simulink model "ex_sdl_flexible_shaft"  (R2022a)
settings: Solver=VariableStepAuto  StartTime=0.0  StopTime=stopTime  RelTol=1e-3  AbsTol=1e-6  EnableMultiTasking=on
InitFcn:
  | % Shaft properties
  | fShaft.Material = 'Aluminum Alloy';
  | fShaft.ShearModulus = 26E9;
  | fShaft.Diameter = 0.025;
  | fShaft.Length = 5;
  | fShaft.Density = 2.7E3;
  | fShaft.DampingCoeff = 0.02;
  | 
  | % Derived properties
  | fShaft.Stiffness = pi/32 * (fShaft.Diameter)^4 ...
  | * fShaft.ShearModulus / fShaft.Length;
  | 
  | fShaft.Inertia = pi/32 * (fShaft.Diameter)^4 ...
  | * fShaft.Density * fShaft.Length ;
values from neighbouring files (symbols this model uses):
  maxPressure = maxPressures(i)    [script1_generate_training_data.m]    (also in script3_test_model.m = maxPressuresTest(i))
undefined symbols (not defined in the file or in its folder): sigbuilder_block
libraries: fl_lib x12, nesl_utility x5, sdl_lib x3
CloseFcn:
  | try,close(h1_sdl_flexible_shaft),end
  | clear h1_sdl_flexible_shaft
  | try,close(h2_sdl_flexible_shaft),end
  | clear h2_sdl_flexible_shaft
  | 
  | 
  | clear simlog_sdl_flexible_shaft
Description:
  | Flexible Shaft
settings Model: FPTRunName=Active  Creator=The MathWorks, Inc.  LastModifiedBy=DNE
settings SolverCC: AutoScaleAbsTol=off  AlgebraicLoopSolver=TrustRegion  MaxZcPerStep=1
settings DataIOCC: LimitDataPoints=on  MaxDataPoints=10000  SaveFormat=Array  SignalLoggingName=logsout_sdl_flexible_shaft
settings OptimizationCC: ExpressionDepthLimit=2147483647  InitFltsAndDblsToZero=on  LifeSpan=inf
settings DebuggingCC: AlgebraicLoopMsg=none  SaveWithParameterizedLinksMsg=none  SignalResolutionControl=TryResolveAllWithWarning  MultiTaskDSMMsg=warning  MultiTaskCondExecSysMsg=none  UnconnectedInputMsg=warning  UnconnectedOutputMsg=warning  UnconnectedLineMsg=warning  StateNameClashWarn=warning  PregeneratedLibrarySubsystemCodeDiagnostic=none  SFUnexpectedBacktrackingDiag=warning  SFNoUnconditionalDefaultTransitionDiag=warning  SFExecutionAtInitializationDiag=none  SFMachineParentedDataDiag=warning  ArithmeticOperatorsInVariantConditions=warning
settings HardwareCC: ProdBitPerPointer=32  ProdBitPerSizeT=32  ProdBitPerPtrDiffT=32  ProdLargestAtomicFloat=None  ProdIntDivRoundTo=Undefined  ProdEndianess=Unspecified  ProdWordSize=32  ProdHWDeviceType=32-bit Generic  TargetBitPerPointer=64  TargetBitPerSizeT=64  TargetBitPerPtrDiffT=64  TargetLongLongMode=on  TargetIntDivRoundTo=Zero  TargetEndianess=LittleEndian  TargetWordSize=64  TargetHWDeviceType=MATLAB Host  ProdEqTarget=off
settings ModelReferenceCC: PropagateSignalLabelsOutOfModel=off
settings SFSimCC: SimUseLocalCustomCode=off  CustomCodeUndefinedFunction=UseInterfaceOnly
settings RTWCC: Description=Generic Real-Time Target  RTWUseLocalCustomCode=off  DLArmComputeVersion=19.05
settings CodeAppCC: StateflowObjectComments=on
settings GRTTargetCC: TargetLangStandard=C89/C90 (ANSI)  CombineOutputUpdateFcns=off  GRTInterface=on
settings ConfigComp: CovMetricSettings=dw  CovSaveCumulativeToWorkspaceVar=on  CovSaveSingleToWorkspaceVar=on  CovExternalEMLEnable=off
settings SimscapeCC: SimscapeLogType=all  SimscapeLogSimulationStatistics=on  SimscapeLogName=simlog_sdl_flexible_shaft  SimscapeLogDataHistory=10000

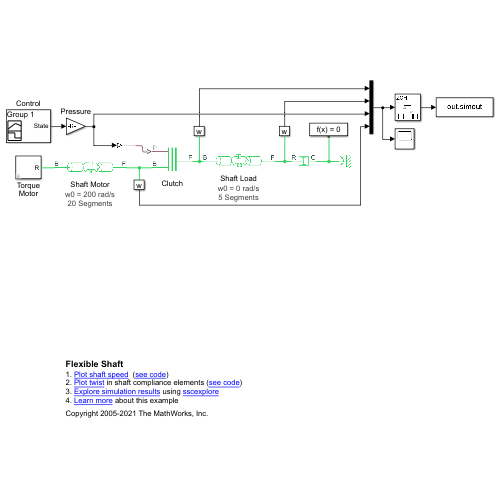
[thumbnail: Simulink's stored preview of the top-level diagram]
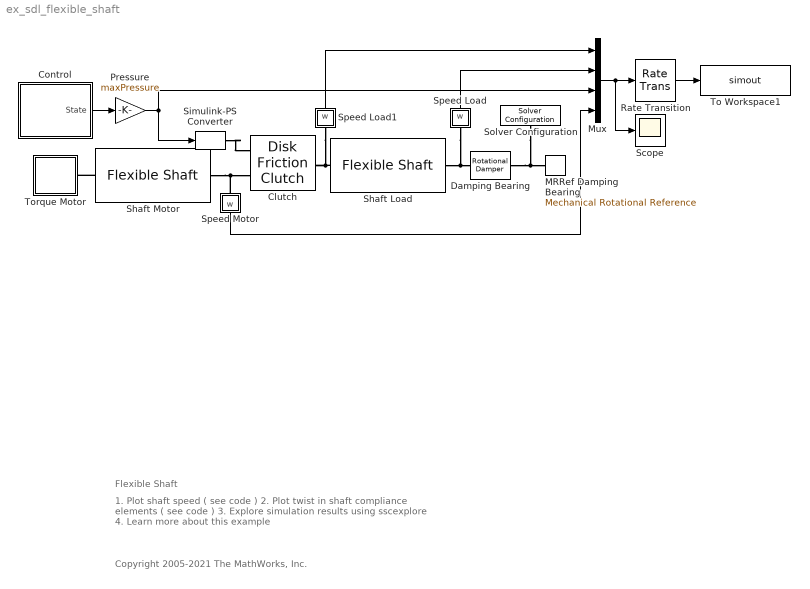
== system ex_sdl_flexible_shaft ==
  note: Flexible Shaft
  note: 1. Plot shaft speed ( see code )
      | 2. Plot twist in shaft compliance elements ( see code )
      | 3. Explore simulation results using sscexplore
      | 4. Learn more about this example
  note: Copyright 2005-2021 The MathWorks, Inc.
  Clutch : sdl_lib/Clutches/Disk Friction Clutch  geometry_model=1  r_eff=40 mm  d_o=150 mm  d_i=100 mm  nS=6  piston_area=0.001 m^2  unidirectional=0  friction_model=1  mu_w_vector=[ 0 0.1 0.2 0.3 0.4 0.5 1 2 5 10 100 1000 ] rad/s  temperature_TLU=[280.0, 300.0, 320.0] K  mu_static=1.1  mu_static_vector=[0.4, 0.38, 0.36]  mu_coulomb=1  mu_coulomb_vector=[ 0.29 0.28 0.26 0.22 0.21 0.2 0.2 0.19 0.19 0.19 0.19 0.19 ]  mu_coulomb_temp_vector=[0.3, 0.28, 0.25]  mu_coulomb_matrix=[0.34, 0.32, 0.3; 0.3, 0.28, 0.25; 0.25, 0.2, 0.15]  mu_interp_method=1  mu_extrap_method=1  d_f=1  w_tol=0.001 rad/s  pressure_min=0 Pa  mu_visc=0 N*m/(rad/s)  initial_state_locked=0  enable_faults=simscape.enum.onoff.off  fault_type=sdl.enum.clutchFault.lock  external_fault=simscape.enum.onoff.off  temporal_fault=simscape.enum.onoff.off  fault_time=5 s  report_fault=simscape.enum.assert.action.none  thermal_mass=25 kJ/K  T_init=300 K
      settings: SourceProductBaseCode=LD  InternalSimscapePortConfiguration="{\"Bottom\":[],\"Left\":[{\"id\":\"P\",\"label\":\"P\",\"type\":\"input\"},{\"id\":\"B\",\"label\":\"B\",\"type\":\"foundation.mechanical.rotational.rotational\"}],\"Right\":[{\"id\":\"F\",\"label\":\"F\",\"type\":\"foundation.mechanical.rotational.rotational\"}],\"Top\":[]}"
  Control : Subsystem  Tag=STV Subsys  LoadFcn=sigbuilder_block('load');  StartFcn=sigbuilder_block('start');  StopFcn=sigbuilder_block('stop');  ClipboardFcn=sigbuilder_block('clipboard');  mask(Sigbuilder block){tuvar=[0:10]}
      mask help: Sigbuilder GUI
      mask init:
      | if ~strcmp(get_param(bdroot(gcbh),'SimulationStatus'),'stopped') tuvar = sigbuilder_block('maskInit'); end
      settings: CopyFcn=sigbuilder_block('copy');  DeleteFcn=sigbuilder_block('delete');  ModelCloseFcn=sigbuilder_block('modelClose');  PreSaveFcn=sigbuilder_block('preSave');  PauseFcn=sigbuilder_block('pause')  ContinueFcn=sigbuilder_block('continue')  NameChangeFcn=sigbuilder_block('namechange');  OpenFcn=sigbuilder_block('open',[320.25 141 457.5 466.5 ]);  CloseFcn=sigbuilder_block('close');
      mask Display: plot(0, 0, 100, 100,[2, 2, 32, 32, 2], [68, 8, 8, 68, 68],[32, 2], [38, 38], [32, 19, 2],[53, 60, 44], [32, 17, 17, 2],[16, 16, 31, 31]);txt = getActiveGroup(gcbh);text(2, 100, txt,'verticalAlignment', 'top');
  Damping Bearing : fl_lib/Mechanical/Rotational Elements/Rotational Damper  D=0.01 N*m/(rad/s)  w_specify=off  w_priority=High  w=0 rad/s  w_nominal_specify=off  w_nominal_unit=rad/s  w_nominal_value=1  t_specify=off  t_priority=High  t=0 N*m  t_nominal_specify=off  t_nominal_unit=N*m  t_nominal_value=1
      settings: SourceProductBaseCode=PW,SS,VE
  MRRef Damping Bearing : fl_lib/Mechanical/Rotational Elements/Mechanical Rotational Reference
      settings: SourceProductBaseCode=PW,SS,VE
  Mux : Mux
  Pressure : Gain  Gain=maxPressure  SaturateOnIntegerOverflow=on  OutDataTypeStr=Inherit: Same as input  ParamDataTypeStr=Inherit: Same as input
  Rate Transition : RateTransition  OutPortSampleTime=timeInterval
  Scope : Scope
  Shaft Load : sdl_lib/Couplings & Drives/Flexible Shaft  modelTransverse=simscape.enum.onoff.off  n_segments=5  parameterization=sdl.enum.shaftParameterization.StiffnessInertia  length=fShaft.Length m  lengths=[1, .5, .25] m  shaft_stiffness=fShaft.Stiffness N*m/rad  shaft_inertia=fShaft.Inertia kg*m^2  shaft_stiffnesses=[400000, 200000, 100000] N*m/rad  shaft_inertias=[.025, .02, .015] kg*m^2  eiIN=5e5 m^4*Pa  rhoaIN=19 kg/m  eiINs=[600000, 500000, 400000] m^4*Pa  rhoaINs=[20, 19, 18] kg/m  density=fShaft.Density kg/m^3  shear_modulus=fShaft.ShearModulus Pa  elastic_modulus=200e9 Pa  shaft_construction=sdl.enum.shaftConstruction.solid  diameter_outer=fShaft.Diameter m  diameter_inner=fShaft.Diameter/2 m  diameter_outers=[.085, .075, .065] m  diameter_inners=[.055, .05, .045] m  damping_ratio=fShaft.DampingCoeff  mu_visc_BF=[0, 0] N*m/(rad/s)  mu_visc=[ 0 0 ] N*m/(rad/s)  initial_deflection=0 rad  initial_velocity=0 rad/s  num_supports=sdl.enum.num_supports.two  z_support=[0, fShaft.Length] m  boundaryB1=sdl.enum.shaftSupport.clamp  DrotB1_row=[100000, 100000] N*m/(rad/s)  DtransB1_row=[200000, -440000, -440000, 3500000] N/(m/s)  DtransB1_w_mat=[200000, -440000, -440000, 3500000; 100000, -250000, -250000, 1400000; 50000, -100000, -100000, 200000] N/(m/s)  KrotB1_row=[10000000, 10000000] N*m/rad  KtransB1_row=[10000000, -2000000, -3000000, 50000000] N/m  KtransB1_w_mat=[10000000, -6000000, -35000000, 80000000; 10000000, -2000000, -3000000, 50000000; 10000000, -500000, -25000000, 30000000] N/m  boundaryI1=sdl.enum.shaftSupport.clamp  DrotI1_row=[100000, 100000] N*m/(rad/s)  DtransI1_row=[200000, -440000, -440000, 3500000] N/(m/s)  DtransI1_w_mat=[200000, -440000, -440000, 3500000; 100000, -250000, -250000, 1400000; 50000, -100000, -100000, 200000] N/(m/s)  KrotI1_row=[10000000, 10000000] N*m/rad  KtransI1_row=[10000000, -2000000, -3000000, 50000000] N/m  KtransI1_w_mat=[10000000, -6000000, -35000000, 80000000; 10000000, -2000000, -3000000, 50000000; 10000000, -500000, -25000000, 30000000] N/m  boundaryI2=sdl.enum.shaftSupport.clamp  DrotI2_row=[100000, 100000] N*m/(rad/s)  DtransI2_row=[200000, -440000, -440000, 3500000] N/(m/s)  DtransI2_w_mat=[200000, -440000, -440000, 3500000; 100000, -250000, -250000, 1400000; 50000, -100000, -100000, 200000] N/(m/s)  KrotI2_row=[10000000, 10000000] N*m/rad  KtransI2_row=[10000000, -2000000, -3000000, 50000000] N/m  KtransI2_w_mat=[10000000, -6000000, -35000000, 80000000; 10000000, -2000000, -3000000, 50000000; 10000000, -500000, -25000000, 30000000] N/m  boundaryF1=sdl.enum.shaftSupport.clamp  DrotF1_row=[100000, 100000] N*m/(rad/s)  DtransF1_row=[200000, -440000, -440000, 3500000] N/(m/s)  DtransF1_w_mat=[200000, -440000, -440000, 3500000; 100000, -250000, -250000, 1400000; 50000, -100000, -100000, 200000] N/(m/s)  KrotF1_row=[10000000, 10000000] N*m/rad  KtransF1_row=[10000000, -2000000, -3000000, 50000000] N/m  KtransF1_w_mat=[10000000, -6000000, -35000000, 80000000; 10000000, -2000000, -3000000, 50000000; 10000000, -500000, -25000000, 30000000] N/m  bearing_speed=[200, 500, 1500] rpm  alpha=10 1/s  beta=1e-8 s  noDisk=sdl.enum.shaftDisks.none  zDisk=0.5 m  mDiskIN=2 kg  IdDiskIN=0.025 kg*m^2  IpDiskIN=0.050 kg*m^2  offsetMR=[.01, .01] m*kg  offsetMassLocation=[.33, .67] m  offsetMR_initialAngleIN=[0, pi] rad  AnalysisMethod=sdl.enum.bendingAnalysisMethod.LumpedMass  ModeInputMethod=sdl.enum.modeInputMethod.SimscapeDetermined  numModesIn=6  mode_speed_dependency=sdl.enum.mode_speed_dependency.Static  OmegaNom=100 rpm  wMax=50000 rad/s  dz=0.01 m  userMode_w=[280, 644, 615, 1285] rad/s  userMode_w_mat=[257, 780, 580, 1560; 280, 644, 615, 1285; 294, 513, 636, 1020] rad/s  userMode_z=[0, .1, .2, .3, .4, .5, .6, .7, .8, .9, 1] m  userMode_shapeX=[.1648, .0086, -.2759, .0162; .1671, .0093, -.2231, .0133; .1691, .01, -.1689, .0102; .1707, .0105, -.1135, .007; .1717, .0108, -.057, .0035; .1721, .0109, 0, 0; .1717, .0108, .057, -.0035; .1707, .0105, .1135, -.007; .1691, .01, .1689, -.0102; .1671, .0093, .2231, -.0133; .1648, .0086, .2759, -.0162]  userMode_shapeX_mat=cat(3, [.1842, .0134, -.3072, .0272; .1863, .0152, -.2482, .0226; .1882, .0169, -.1878, .0176; .1897, .0182, -.1261, .0121; .1906, .019, -.0634, .0062; .191, .0193, 0, 0; .1906, .019, .0634, -.0062; .1897, .0182, .1261, -.0121; .1882, .0169, .1878, -.0176; .1863, .0152, .2482, -.0226; .1842, .0134, .3072, -.0272], [.1648, .0086, -.2759, .0162; .1671, .0093, -.2231, .0133; .1691, .01, -.1689, .0102; .1707, .0105, -.1135, .007; .1717, .0108, -.057, .0035; .1721, .0109, 0, 0; .1717, .0108, .057, -.0035; .1707, .0105, .1135, -.007; .1691, .01, .1689, -.0102; .1671, .0093, .2231, -.0133; .1648, .0086, .2759, -.0162], [.1291, .0046, -.2166, .0082; .131, .0048, -.1751, .0067; .1327, .005, -.1327, .0051; .1341, .0052, -.0891, .0035; .135, .0053, -.0448, .0017; .1353, .0053, 0, 0; .135, .0053, .0448, -.0017; .1341, .0052, .0891, -.0035; .1327, .005, .1327, -.0051; .131, .0048, .1751, -.0067; .1291, .0046, .2166, -.0082])  userMode_shapeY=[.1193, -.1784, -.1997, -.3348; .1209, -.1933, -.1615, -.2751; .1224, -.2068, -.1223, -.2119; .1235, -.2176, -.0821, -.1445; .1243, -.2245, -.0413, -.0734; .1246, -.2269, 0, 0; .1243, -.2245, .0413, .0734; .1235, -.2176, .0821, .1445; .1224, -.2068, .1223, .2119; .1209, -.1933, .1615, .2751; .1193, -.1784, .1997, .3348]  userMode_shapeY_mat=cat(3, [.0885, -.1625, -.1475, -.3301; .0895, -.1847, -.1192, -.2745; .0904, -.2048, -.0902, -.2141; .0911, -.2209, -.0606, -.1475; .0916, -.2313, -.0304, -.0754; .0917, -.2349, 0, 0; .0916, -.2313, .0304, .0754; .0911, -.2209, .0606, .1475; .0904, -.2048, .0902, .2141; .0895, -.1847, .1192, .2745; .0885, -.1625, .1475, .3301], [.1193, -.1784, -.1997, -.3348; .1209, -.1933, -.1615, -.2751; .1224, -.2068, -.1223, -.2119; .1235, -.2176, -.0821, -.1445; .1243, -.2245, -.0413, -.0734; .1246, -.2269, 0, 0; .1243, -.2245, .0413, .0734; .1235, -.2176, .0821, .1445; .1224, -.2068, .1223, .2119; .1209, -.1933, .1615, .2751; .1193, -.1784, .1997, .3348], [.1566, -.1901, -.2628, -.3377; .1589, -.1994, -.2125, -.2753; .161, -.2079, -.1609, -.2103; .1627, -.2146, -.1081, -.1424; .1638, -.219, -.0544, -.0719; .1642, -.2205, 0, 0; .1638, -.219, .0544, .0719; .1627, -.2146, .1081, .1424; .161, -.2079, .1609, .2103; .1589, -.1994, .2125, .2753; .1566, -.1901, .2628, .3377])
      settings: SourceProductBaseCode=LD  InternalSimscapePortConfiguration="{\"Bottom\":[],\"Left\":[{\"id\":\"B\",\"label\":\"B\",\"type\":\"foundation.mechanical.rotational.rotational\"}],\"Right\":[{\"id\":\"F\",\"label\":\"F\",\"type\":\"foundation.mechanical.rotational.rotational\"}],\"Top\":[]}"
      settings: AttributesFormatString=|
      | w0 = %<initial_velocity> %<initial_velocity_unit>
      | %<n_segments> Segments
  Shaft Motor : sdl_lib/Couplings & Drives/Flexible Shaft  modelTransverse=simscape.enum.onoff.off  n_segments=20  parameterization=sdl.enum.shaftParameterization.MaterialProperties  length=fShaft.Length m  lengths=[1, .5, .25] m  shaft_stiffness=fShaft.Stiffness N*m/rad  shaft_inertia=fShaft.Inertia kg*m^2  shaft_stiffnesses=[400000, 200000, 100000] N*m/rad  shaft_inertias=[.025, .02, .015] kg*m^2  eiIN=5e5 m^4*Pa  rhoaIN=19 kg/m  eiINs=[600000, 500000, 400000] m^4*Pa  rhoaINs=[20, 19, 18] kg/m  density=fShaft.Density kg/m^3  shear_modulus=fShaft.ShearModulus Pa  elastic_modulus=200e9 Pa  shaft_construction=sdl.enum.shaftConstruction.annular  diameter_outer=fShaft.Diameter m  diameter_inner=fShaft.Diameter/2 m  diameter_outers=[.085, .075, .065] m  diameter_inners=[.055, .05, .045] m  damping_ratio=fShaft.DampingCoeff  mu_visc_BF=[0, 0] N*m/(rad/s)  mu_visc=[ 0 0 ] N*m/(rad/s)  initial_deflection=0 rad  initial_velocity=200 rad/s  num_supports=sdl.enum.num_supports.two  z_support=[0, fShaft.Length] m  boundaryB1=sdl.enum.shaftSupport.clamp  DrotB1_row=[1000, 1000] N*m/(rad/s)  DtransB1_row=[20000, -44000, -44000, 350000] N/(m/s)  DtransB1_w_mat=[200000, -440000, -440000, 3500000; 100000, -250000, -250000, 1400000; 50000, -100000, -100000, 200000] N/(m/s)  KrotB1_row=[10000, 10000] N*m/rad  KtransB1_row=[1000000, -200000, -300000, 5000000] N/m  KtransB1_w_mat=[10000000, -6000000, -35000000, 80000000; 10000000, -2000000, -3000000, 50000000; 10000000, -500000, -25000000, 30000000] N/m  boundaryI1=sdl.enum.shaftSupport.clamp  DrotI1_row=[100000, 100000] N*m/(rad/s)  DtransI1_row=[200000, -440000, -440000, 3500000] N/(m/s)  DtransI1_w_mat=[200000, -440000, -440000, 3500000; 100000, -250000, -250000, 1400000; 50000, -100000, -100000, 200000] N/(m/s)  KrotI1_row=[10000000, 10000000] N*m/rad  KtransI1_row=[10000000, -2000000, -3000000, 50000000] N/m  KtransI1_w_mat=[10000000, -6000000, -35000000, 80000000; 10000000, -2000000, -3000000, 50000000; 10000000, -500000, -25000000, 30000000] N/m  boundaryI2=sdl.enum.shaftSupport.clamp  DrotI2_row=[100000, 100000] N*m/(rad/s)  DtransI2_row=[200000, -440000, -440000, 3500000] N/(m/s)  DtransI2_w_mat=[200000, -440000, -440000, 3500000; 100000, -250000, -250000, 1400000; 50000, -100000, -100000, 200000] N/(m/s)  KrotI2_row=[10000000, 10000000] N*m/rad  KtransI2_row=[10000000, -2000000, -3000000, 50000000] N/m  KtransI2_w_mat=[10000000, -6000000, -35000000, 80000000; 10000000, -2000000, -3000000, 50000000; 10000000, -500000, -25000000, 30000000] N/m  boundaryF1=sdl.enum.shaftSupport.clamp  DrotF1_row=[1000, 1000] N*m/(rad/s)  DtransF1_row=[20000, -44000, -44000, 350000] N/(m/s)  DtransF1_w_mat=[200000, -440000, -440000, 3500000; 100000, -250000, -250000, 1400000; 50000, -100000, -100000, 200000] N/(m/s)  KrotF1_row=[10000, 10000] N*m/rad  KtransF1_row=[1000000, -200000, -300000, 5000000] N/m  KtransF1_w_mat=[10000000, -6000000, -35000000, 80000000; 10000000, -2000000, -3000000, 50000000; 10000000, -500000, -25000000, 30000000] N/m  bearing_speed=[200, 500, 1500] rpm  alpha=10 1/s  beta=1e-8 s  noDisk=sdl.enum.shaftDisks.none  zDisk=0.5 m  mDiskIN=2 kg  IdDiskIN=0.025 kg*m^2  IpDiskIN=0.050 kg*m^2  offsetMR=[.01, .01] m*kg  offsetMassLocation=[.33, .67] m  offsetMR_initialAngleIN=[0, pi] rad  AnalysisMethod=sdl.enum.bendingAnalysisMethod.LumpedMass  ModeInputMethod=sdl.enum.modeInputMethod.SimscapeDetermined  numModesIn=6  mode_speed_dependency=sdl.enum.mode_speed_dependency.Static  OmegaNom=100 rpm  wMax=50000 rad/s  dz=0.01 m  userMode_w=[162, 162, 649, 649, 1460, 1460, 2596, 2596] rad/s  userMode_w_mat=[257, 780, 580, 1560; 280, 644, 615, 1285; 294, 513, 636, 1020] rad/s  userMode_z=[0, .1, .2, .3, .4, .5, .6, .7, .8, .9, 1] m  userMode_shapeX=[.1648, .0086, -.2759, .0162; .1671, .0093, -.2231, .0133; .1691, .01, -.1689, .0102; .1707, .0105, -.1135, .007; .1717, .0108, -.057, .0035; .1721, .0109, 0, 0; .1717, .0108, .057, -.0035; .1707, .0105, .1135, -.007; .1691, .01, .1689, -.0102; .1671, .0093, .2231, -.0133; .1648, .0086, .2759, -.0162]  userMode_shapeX_mat=cat(3, [.1842, .0134, -.3072, .0272; .1863, .0152, -.2482, .0226; .1882, .0169, -.1878, .0176; .1897, .0182, -.1261, .0121; .1906, .019, -.0634, .0062; .191, .0193, 0, 0; .1906, .019, .0634, -.0062; .1897, .0182, .1261, -.0121; .1882, .0169, .1878, -.0176; .1863, .0152, .2482, -.0226; .1842, .0134, .3072, -.0272], [.1648, .0086, -.2759, .0162; .1671, .0093, -.2231, .0133; .1691, .01, -.1689, .0102; .1707, .0105, -.1135, .007; .1717, .0108, -.057, .0035; .1721, .0109, 0, 0; .1717, .0108, .057, -.0035; .1707, .0105, .1135, -.007; .1691, .01, .1689, -.0102; .1671, .0093, .2231, -.0133; .1648, .0086, .2759, -.0162], [.1291, .0046, -.2166, .0082; .131, .0048, -.1751, .0067; .1327, .005, -.1327, .0051; .1341, .0052, -.0891, .0035; .135, .0053, -.0448, .0017; .1353, .0053, 0, 0; .135, .0053, .0448, -.0017; .1341, .0052, .0891, -.0035; .1327, .005, .1327, -.0051; .131, .0048, .1751, -.0067; .1291, .0046, .2166, -.0082])  userMode_shapeY=[.1193, -.1784, -.1997, -.3348; .1209, -.1933, -.1615, -.2751; .1224, -.2068, -.1223, -.2119; .1235, -.2176, -.0821, -.1445; .1243, -.2245, -.0413, -.0734; .1246, -.2269, 0, 0; .1243, -.2245, .0413, .0734; .1235, -.2176, .0821, .1445; .1224, -.2068, .1223, .2119; .1209, -.1933, .1615, .2751; .1193, -.1784, .1997, .3348]  userMode_shapeY_mat=cat(3, [.0885, -.1625, -.1475, -.3301; .0895, -.1847, -.1192, -.2745; .0904, -.2048, -.0902, -.2141; .0911, -.2209, -.0606, -.1475; .0916, -.2313, -.0304, -.0754; .0917, -.2349, 0, 0; .0916, -.2313, .0304, .0754; .0911, -.2209, .0606, .1475; .0904, -.2048, .0902, .2141; .0895, -.1847, .1192, .2745; .0885, -.1625, .1475, .3301], [.1193, -.1784, -.1997, -.3348; .1209, -.1933, -.1615, -.2751; .1224, -.2068, -.1223, -.2119; .1235, -.2176, -.0821, -.1445; .1243, -.2245, -.0413, -.0734; .1246, -.2269, 0, 0; .1243, -.2245, .0413, .0734; .1235, -.2176, .0821, .1445; .1224, -.2068, .1223, .2119; .1209, -.1933, .1615, .2751; .1193, -.1784, .1997, .3348], [.1566, -.1901, -.2628, -.3377; .1589, -.1994, -.2125, -.2753; .161, -.2079, -.1609, -.2103; .1627, -.2146, -.1081, -.1424; .1638, -.219, -.0544, -.0719; .1642, -.2205, 0, 0; .1638, -.219, .0544, .0719; .1627, -.2146, .1081, .1424; .161, -.2079, .1609, .2103; .1589, -.1994, .2125, .2753; .1566, -.1901, .2628, .3377])
      settings: SourceProductBaseCode=LD  InternalSimscapePortConfiguration="{\"Bottom\":[],\"Left\":[{\"id\":\"B\",\"label\":\"B\",\"type\":\"foundation.mechanical.rotational.rotational\"}],\"Right\":[{\"id\":\"F\",\"label\":\"F\",\"type\":\"foundation.mechanical.rotational.rotational\"}],\"Top\":[]}"
      settings: AttributesFormatString=|
      | w0 = %<initial_velocity> %<initial_velocity_unit>
      | %<n_segments> Segments
  Simulink-PS Converter : nesl_utility/Simulink-PS Converter  PhysicalDomain=network_engine_domain  SubClassName=ps_input  LeftPortType=input  RightPortType=output  PseudoPeriodic=off  Frequencies=[]  NoiseDistribution=none  NoiseParameters=[]  Unit=Pa  AffineConversion=off  FilteringAndDerivatives=zero  SimscapeFilterOrder=1  InputFilterTimeConstant=.001  UdotUserProvided=0
      settings: SourceProductBaseCode=SS,PW,VE
  Solver Configuration : nesl_utility/Solver Configuration  PhysicalDomain=network_engine_domain  SubClassName=solver  LeftPortType=input  RightPortType=generic  Tones=[]  Harmonics=[]  SimulateNoise=off  Profile=off  UseLocalSampling=off  EnableSwitchedLinearOptims=on  FrequencyDomain=off  UseCCode=off  RelTol=0.001  AbsTol=1e-06  MinStep=1e-09  ToWorkspace=off  RevertToSquareIcSolve=off  NumHomotopyIterations=100  PhasorMode=off  PhasorModeNumHarmonics=1  IndexReductionMethod=DerivativeReplacement  DoDC=off  ResidualTolerance=1e-9  UseLocalSolver=off  LocalSolverChoice=NE_PARTITIONING_ADVANCER  LocalSolverSampleTime=.0001  DoFixedCost=off  MaxNonlinIter=3  MaxModeIter=2  ComputeImpulses=off  ImpulseIterations=2  LinearAlgebra=auto  LinearAlgebraNumThread=0  EquationFormulation=NE_TIME_EF  DelaysMemoryBudget=1024  AutomaticFiltering=on  FilteringTimeConstant=0.001  PartitionStorageMethod=EXHAUSTIVE  PartitionMemoryBudget=1024  PartitionMethod=ROBUST
      settings: SourceProductBaseCode=SS,PW,VE
  Speed Load : Subsystem
      mask Display: disp('w')
  Speed Load1 : Subsystem
      mask Display: disp('w')
  Speed Motor : Subsystem
      mask Display: disp('w')
  To Workspace1 : ToWorkspace  VariableName=simout  SaveFormat=Timeseries  SampleTime=-1
  Torque Motor : Subsystem  mask(Constant Torque Motor){motorTorque=20, bearingD=0.1}
      mask prompts: motorTorque "Demanded torque (Nm)"; bearingD "Bearing damping ( Nm/(rad/s) )"
      mask help:
      | Models a simple constant torque motor with bearing loss.
      |
      | OutputTorque = DemandedTorque - BearingDamping * RotationalSpeed
  wires:
  Pressure/1 -> Mux/3, Simulink-PS Converter/1
  Mux/1 -> Scope/1, Rate Transition/1
  Rate Transition/1 -> To Workspace1/1
  Speed Load1/1(w) -> Mux/1
  Speed Load/1(w) -> Mux/2
  Control/1(State) -> Pressure/1
  Speed Motor/1(w) -> Mux/4
  connections:
  Shaft Motor/LConn1 -- Torque Motor/LConn1
  Shaft Load/RConn1 -- Speed Load/LConn1 -- Damping Bearing/LConn1
  Damping Bearing/RConn1 -- Solver Configuration/RConn1 -- MRRef Damping Bearing/LConn1
  Shaft Load/LConn1 -- Speed Load1/LConn1 -- Clutch/RConn1
  Shaft Motor/RConn1 -- Speed Motor/LConn1 -- Clutch/LConn2
  Simulink-PS Converter/RConn1 -- Clutch/LConn1

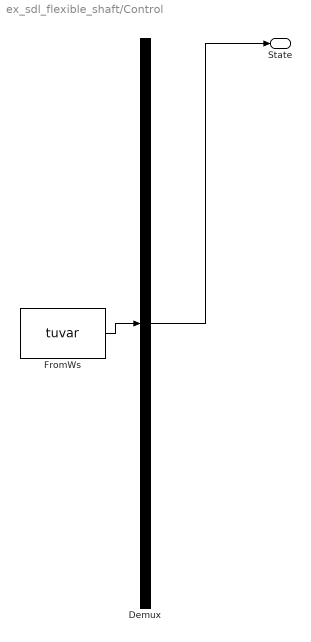
== system ex_sdl_flexible_shaft/Control ==
  Demux : Demux  Tag=STV Demux  Outputs=1
      settings: DisplayOption=none
  FromWs : FromWorkspace  Tag=STV FromWs  VariableName=tuvar
      SigBuilderData=|
      | common.afterFinalStr = 'Extrapolate'
      | common.sampleTime = 0
      | dataSet.timeRange = [0 0.4]
      | dataSet.name = 'Group 1'
      | sbobj.Name = 'Signal Builder'
      | sbobj.Groups.Name = 'Group 1'
      | sbobj.Groups.Signals.Name = 'State'
      | sbobj.Groups.Signals.XData = [0 0.01 0.06 0.075 0.1 0.4]
      | sbobj.Groups.Signals.YData = [0 0 1 1 0 0]
      | sbobj.Groups.TimeRange = [0 0.4]
  State : Outport  Tag=STV Outport  VectorParamsAs1DForOutWhenUnconnected=off
  wires:
  Demux/1 -> State/1
  FromWs/1 -> Demux/1

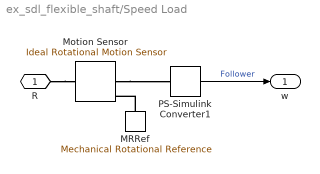
== system ex_sdl_flexible_shaft/Speed Load ==
  MRRef : fl_lib/Mechanical/Rotational Elements/Mechanical Rotational Reference
      settings: SourceProductBaseCode=PW,SS,VE
  Motion Sensor : fl_lib/Mechanical/Mechanical Sensors/Ideal Rotational Motion Sensor  wrap_angle=simscape.enum.onoff.off  offset=0 rad
      settings: SourceProductBaseCode=PW,SS,VE
  PS-Simulink Converter1 : nesl_utility/PS-Simulink Converter  PhysicalDomain=network_engine_domain  SubClassName=ps_output  LeftPortType=input  RightPortType=output  PseudoPeriodic=off  Frequencies=[]  VectorFormat=1-D array  Unit=rad/s  AffineConversion=off
      settings: SourceProductBaseCode=SS,PW,VE
  R : PMIOPort  Side=Left
  w : Outport  VectorParamsAs1DForOutWhenUnconnected=off
  wires:
  PS-Simulink Converter1/1 -> w/1  "Follower"
  connections:
  R/RConn1 -- Motion Sensor/LConn1
  Motion Sensor/RConn2 -- PS-Simulink Converter1/LConn1
  MRRef/LConn1 -- Motion Sensor/RConn1

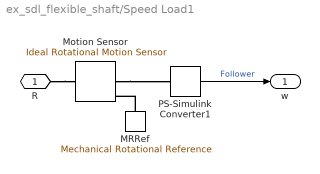
== system ex_sdl_flexible_shaft/Speed Load1 ==
  MRRef : fl_lib/Mechanical/Rotational Elements/Mechanical Rotational Reference
      settings: SourceProductBaseCode=PW,SS,VE
  Motion Sensor : fl_lib/Mechanical/Mechanical Sensors/Ideal Rotational Motion Sensor  wrap_angle=simscape.enum.onoff.off  offset=0 rad
      settings: SourceProductBaseCode=PW,SS,VE
  PS-Simulink Converter1 : nesl_utility/PS-Simulink Converter  PhysicalDomain=network_engine_domain  SubClassName=ps_output  LeftPortType=input  RightPortType=output  PseudoPeriodic=off  Frequencies=[]  VectorFormat=1-D array  Unit=rad/s  AffineConversion=off
      settings: SourceProductBaseCode=SS,PW,VE
  R : PMIOPort  Side=Left
  w : Outport  VectorParamsAs1DForOutWhenUnconnected=off
  wires:
  PS-Simulink Converter1/1 -> w/1  "Follower"
  connections:
  R/RConn1 -- Motion Sensor/LConn1
  Motion Sensor/RConn2 -- PS-Simulink Converter1/LConn1
  MRRef/LConn1 -- Motion Sensor/RConn1

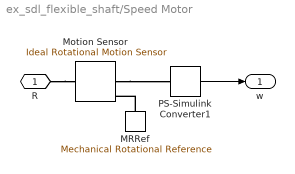
== system ex_sdl_flexible_shaft/Speed Motor ==
  MRRef : fl_lib/Mechanical/Rotational Elements/Mechanical Rotational Reference
      settings: SourceProductBaseCode=PW,SS,VE
  Motion Sensor : fl_lib/Mechanical/Mechanical Sensors/Ideal Rotational Motion Sensor  wrap_angle=simscape.enum.onoff.off  offset=0 rad
      settings: SourceProductBaseCode=PW,SS,VE
  PS-Simulink Converter1 : nesl_utility/PS-Simulink Converter  PhysicalDomain=network_engine_domain  SubClassName=ps_output  LeftPortType=input  RightPortType=output  PseudoPeriodic=off  Frequencies=[]  VectorFormat=1-D array  Unit=rad/s  AffineConversion=off
      settings: SourceProductBaseCode=SS,PW,VE
  R : PMIOPort  Side=Left
  w : Outport  VectorParamsAs1DForOutWhenUnconnected=off
  wires:
  PS-Simulink Converter1/1 -> w/1
  connections:
  MRRef/LConn1 -- Motion Sensor/RConn1
  Motion Sensor/RConn2 -- PS-Simulink Converter1/LConn1
  R/RConn1 -- Motion Sensor/LConn1

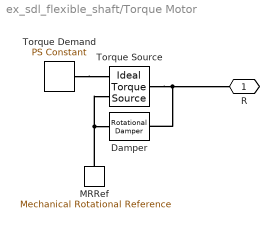
== system ex_sdl_flexible_shaft/Torque Motor ==
  Damper : fl_lib/Mechanical/Rotational Elements/Rotational Damper  D=bearingD N*m/(rad/s)  w_specify=off  w_priority=High  w=0 rad/s  w_nominal_specify=off  w_nominal_unit=rad/s  w_nominal_value=1  t_specify=off  t_priority=High  t=0 N*m  t_nominal_specify=off  t_nominal_unit=N*m  t_nominal_value=1
      settings: SourceProductBaseCode=PW,SS,VE
  MRRef : fl_lib/Mechanical/Rotational Elements/Mechanical Rotational Reference
      settings: SourceProductBaseCode=PW,SS,VE
  Torque Demand : fl_lib/Physical Signals/Sources/PS Constant  constant=motorTorque
      settings: SourceProductBaseCode=PW,SS,VE
  Torque Source : fl_lib/Mechanical/Mechanical Sources/Ideal Torque Source
      settings: SourceProductBaseCode=PW,SS,VE
  R : PMIOPort  Side=Left
  connections:
  Torque Source/LConn1 -- R/RConn1 -- Damper/LConn1
  MRRef/LConn1 -- Torque Source/RConn2 -- Damper/RConn1
  Torque Demand/RConn1 -- Torque Source/RConn1
